simulink model "feedback_control"  (R2020b)
settings: Solver=FixedStepDiscrete  StartTime=0.0  StopTime=inf  FixedStep=T_sample_control  RelTol=1e-3
undefined symbols (not defined in the file): T_sample_control
settings Model: DataDictionary=pid.sldd  EnableAccessToBaseWorkspace=off  ModifiedByFormat=The MathWorks Inc.  SILPILModeSetting=veronly  ExtModeTrigDuration=2  Creator=The MathWorks, Inc.  LastModifiedBy=The MathWorks Inc.
settings DataIOCC: SaveFormat=Array  ReturnWorkspaceOutputs=off
settings OptimizationCC: DefaultParameterBehavior=Inlined  InlineInvariantSignals=on  PassReuseOutputArgsAs=Individual arguments  ExpressionDepthLimit=2147483647  EfficientFloat2IntCast=on  LifeSpan=1  EfficientTunableParamExpr=on
settings DebuggingCC: SolverPrmCheckMsg=warning  FcnCallInpInsideContextMsg=warning  UniqueDataStoreMsg=error  AssertControl=DisableAll  AllowSymbolicDim=off  StateNameClashWarn=warning  StrictBusMsg=ErrorOnBusTreatedAsVector  SFUnexpectedBacktrackingDiag=warning  SFNoUnconditionalDefaultTransitionDiag=warning  SFExecutionAtInitializationDiag=none  ArithmeticOperatorsInVariantConditions=warning
settings HardwareCC: ProdBitPerPointer=32  ProdBitPerSizeT=32  ProdBitPerPtrDiffT=32  ProdLargestAtomicInteger=Long  ProdLargestAtomicFloat=Double  ProdWordSize=32  ProdHWDeviceType=ARM Compatible->ARM Cortex-M
settings ModelReferenceCC: PropagateSignalLabelsOutOfModel=off
settings SFSimCC: SimUseLocalCustomCode=off  CustomCodeUndefinedFunction=UseInterfaceOnly
settings RTWCC: Description=Embedded Coder  SystemTargetFile=ert.tlc  GenCodeOnly=on  TemplateMakefile=ert_default_tmf  GenerateReport=on  RTWUseLocalCustomCode=off  BuildConfiguration=Faster Runs  IncludeHyperlinkInReport=on  LaunchReport=on  GenerateTraceInfo=on  GenerateTraceReport=on  GenerateTraceReportSl=on  GenerateTraceReportSf=on  GenerateTraceReportEml=on  GenerateCodeMetricsReport=on
settings CodeAppCC: IgnoreCustomStorageClasses=off  IgnoreTestpoints=on  CustomSymbolStrType=$N$R$M  StateflowObjectComments=on  InternalIdentifier=Classic
settings ERTTargetCC: MultiwordLength=2048  GenerateSampleERTMain=on  CodeInterfacePackaging=Reusable function  SupportNonFinite=off  ParenthesesLevel=Maximum  InlinedParameterPlacement=NonHierarchical  ERTCustomFileTemplate=example_file_process.tlc  ERTFilePackagingFormat=Compact  ConvertIfToSwitch=off  SuppressUnreachableDefaultCases=off
settings ConfigComp: CovMetricSettings=dw  CovSaveCumulativeToWorkspaceVar=on  CovSaveSingleToWorkspaceVar=on  CovExternalEMLEnable=off  CovSFcnEnable=off

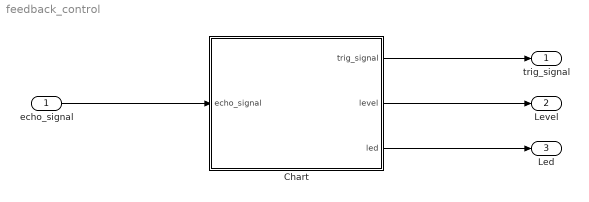
== system feedback_control ==
  echo_signal : Inport  OutDataTypeStr=boolean  PortDimensions=1  SampleTime=T_sample_control
  Chart : Stateflow chart  TreatAsAtomicUnit=on
  trig_signal : Outport  OutDataTypeStr=boolean  PortDimensions=1  SampleTime=T_sample_control
  Level : Outport  Port=2  OutDataTypeStr=uint16
  Led : Outport  Port=3  OutDataTypeStr=boolean
  wires:
  Chart/1(trig_signal) -> trig_signal/1
  Chart/2(level) -> Level/1
  Chart/3(led) -> Led/1
  echo_signal/1 -> Chart/1(echo_signal)

== stateflow chart feedback_control/Chart ==
  state PROCESSING_LOGIC [parallel]
    settings: executionOrder=1
    state TRIG_SIGNAL_ON
      entry:
      trig_signal = true;
    state TRIG_SIGNAL_OFF
      entry:
      trig_signal = false;
      echo_up_check = false;
      exit:
      if echo_up_check == false
      level = 0;
      end
      state ECHO_UP
        entry, during:
        echo_pulse_duration_us = temporalCount(usec);
        exit:
        measures(index) = (echo_pulse_duration_us) / 58;
        level = uint16(sum(measures) / 4);
        index = index + 1;
        if index > 4
        index = 1;
        end
      state ECHO_DOWN
      (default) -> ECHO_DOWN
      ECHO_UP -> ECHO_DOWN : [echo_signal == false]
      ECHO_DOWN -> ECHO_UP : [echo_signal == true]{echo_up_check = true;}
    (default) -> TRIG_SIGNAL_ON
    TRIG_SIGNAL_ON -> TRIG_SIGNAL_OFF : after(20,usec)
    TRIG_SIGNAL_OFF -> TRIG_SIGNAL_ON : after(60,msec)
  state MONITORING_LOGIC [parallel]
    settings: executionOrder=2
    state BLINK_OUTRANGE
      frequency = 0.5;
      state LED_OFF
        entry:
        led = false;
      state LED_ON
        entry:
        led = true;
      (default) -> MONITORING_LOGIC.BLINK_OUTRANGE.LED_ON
      MONITORING_LOGIC.BLINK_OUTRANGE.LED_ON -> MONITORING_LOGIC.BLINK_OUTRANGE.LED_OFF : after(frequency/2, sec)
      MONITORING_LOGIC.BLINK_OUTRANGE.LED_OFF -> MONITORING_LOGIC.BLINK_OUTRANGE.LED_ON : after(frequency/2, sec)
    state BLINK_INRANGE
      frequency = 0.1;
      state LED_OFF
        entry:
        led = false;
      state LED_ON
        entry:
        led = true;
      (default) -> MONITORING_LOGIC.BLINK_INRANGE.LED_ON
      MONITORING_LOGIC.BLINK_INRANGE.LED_OFF -> MONITORING_LOGIC.BLINK_INRANGE.LED_ON : after(frequency - ((single(level)*frequency)/100), sec)
      MONITORING_LOGIC.BLINK_INRANGE.LED_ON -> MONITORING_LOGIC.BLINK_INRANGE.LED_OFF : after((single(level)*frequency)/100, sec)
    state DISCONNECTED_SENSOR
      frequency = 1;
      state LED_OFF
        entry:
        led = false;
      state LED_ON
        entry:
        led = true;
      (default) -> MONITORING_LOGIC.DISCONNECTED_SENSOR.LED_ON
      MONITORING_LOGIC.DISCONNECTED_SENSOR.LED_ON -> MONITORING_LOGIC.DISCONNECTED_SENSOR.LED_OFF : after(frequency/2, sec)
      MONITORING_LOGIC.DISCONNECTED_SENSOR.LED_OFF -> MONITORING_LOGIC.DISCONNECTED_SENSOR.LED_ON : after(frequency/2, sec)
    BLINK_OUTRANGE -> BLINK_INRANGE [order 1] : [level >=10 && level <=100]
    BLINK_INRANGE -> BLINK_OUTRANGE : [level < 10 || level >100]
    (default) -> DISCONNECTED_SENSOR
    (junction 156) -> BLINK_OUTRANGE
    BLINK_OUTRANGE -> (junction 136) [order 2] : [level == 0]
    (junction 174) -> BLINK_INRANGE
    (junction 136) -> DISCONNECTED_SENSOR
    DISCONNECTED_SENSOR -> (junction 174) [order 2] : [level >=10 && level <=100]
    DISCONNECTED_SENSOR -> (junction 156) [order 1] : [level ~= 0 && (level < 10 || level >100)]
  data: echo_signal input boolean; trig_signal output boolean; level output uint16 =uint16(0); measures local double size=4 =[0;0;0;0]; index local uint8 =uint8(1); echo_pulse_duration_us local double; led output boolean; frequency local single; echo_up_check local boolean
